simulink model "sequentialProcessorNarenKolli"  (R2018b)
settings: Solver=VariableStepAuto  StartTime=0.0  StopTime=10  RelTol=1e-3
libraries: hdlsllib x172, simulink_extras x9
(part 4 of 4)

== system sequentialProcessorNarenKolli/8-Bit_Processor /8-Bit_Multiplier/First 8-Bit_Adder/Full Adder5/Half Adder ==
  A : Inport
  B : Inport  Port=2
  AND (calculates carry) : Logic  AllPortsSameDT=off  OutDataTypeStr=boolean
  XOR (calculates sum) : Logic  Operator=XOR  AllPortsSameDT=off  OutDataTypeStr=boolean
  Sum : Outport
  Carry : Outport  Port=2
  wires:
  XOR (calculates sum)/1 -> Sum/1
  B/1 -> XOR (calculates sum)/2, AND (calculates carry)/2
  A/1 -> AND (calculates carry)/1, XOR (calculates sum)/1
  AND (calculates carry)/1 -> Carry/1

== system sequentialProcessorNarenKolli/8-Bit_Processor /8-Bit_Multiplier/First 8-Bit_Adder/Full Adder5/Half Adder1 ==
  A : Inport
  B : Inport  Port=2
  AND (calculates carry) : Logic  AllPortsSameDT=off  OutDataTypeStr=boolean
  XOR (calculates sum) : Logic  Operator=XOR  AllPortsSameDT=off  OutDataTypeStr=boolean
  Sum : Outport
  Carry : Outport  Port=2
  wires:
  XOR (calculates sum)/1 -> Sum/1
  B/1 -> XOR (calculates sum)/2, AND (calculates carry)/2
  A/1 -> AND (calculates carry)/1, XOR (calculates sum)/1
  AND (calculates carry)/1 -> Carry/1

== system sequentialProcessorNarenKolli/8-Bit_Processor /8-Bit_Multiplier/First 8-Bit_Adder/Full Adder6/Half Adder ==
  A : Inport
  B : Inport  Port=2
  AND (calculates carry) : Logic  AllPortsSameDT=off  OutDataTypeStr=boolean
  XOR (calculates sum) : Logic  Operator=XOR  AllPortsSameDT=off  OutDataTypeStr=boolean
  Sum : Outport
  Carry : Outport  Port=2
  wires:
  XOR (calculates sum)/1 -> Sum/1
  B/1 -> XOR (calculates sum)/2, AND (calculates carry)/2
  A/1 -> AND (calculates carry)/1, XOR (calculates sum)/1
  AND (calculates carry)/1 -> Carry/1

== system sequentialProcessorNarenKolli/8-Bit_Processor /8-Bit_Multiplier/First 8-Bit_Adder/Full Adder6/Half Adder1 ==
  A : Inport
  B : Inport  Port=2
  AND (calculates carry) : Logic  AllPortsSameDT=off  OutDataTypeStr=boolean
  XOR (calculates sum) : Logic  Operator=XOR  AllPortsSameDT=off  OutDataTypeStr=boolean
  Sum : Outport
  Carry : Outport  Port=2
  wires:
  XOR (calculates sum)/1 -> Sum/1
  B/1 -> XOR (calculates sum)/2, AND (calculates carry)/2
  A/1 -> AND (calculates carry)/1, XOR (calculates sum)/1
  AND (calculates carry)/1 -> Carry/1

== system sequentialProcessorNarenKolli/8-Bit_Processor /8-Bit_Multiplier/First 8-Bit_Adder/Full Adder7/Half Adder ==
  A : Inport
  B : Inport  Port=2
  AND (calculates carry) : Logic  AllPortsSameDT=off  OutDataTypeStr=boolean
  XOR (calculates sum) : Logic  Operator=XOR  AllPortsSameDT=off  OutDataTypeStr=boolean
  Sum : Outport
  Carry : Outport  Port=2
  wires:
  XOR (calculates sum)/1 -> Sum/1
  B/1 -> XOR (calculates sum)/2, AND (calculates carry)/2
  A/1 -> AND (calculates carry)/1, XOR (calculates sum)/1
  AND (calculates carry)/1 -> Carry/1

== system sequentialProcessorNarenKolli/8-Bit_Processor /8-Bit_Multiplier/First 8-Bit_Adder/Full Adder7/Half Adder1 ==
  A : Inport
  B : Inport  Port=2
  AND (calculates carry) : Logic  AllPortsSameDT=off  OutDataTypeStr=boolean
  XOR (calculates sum) : Logic  Operator=XOR  AllPortsSameDT=off  OutDataTypeStr=boolean
  Sum : Outport
  Carry : Outport  Port=2
  wires:
  XOR (calculates sum)/1 -> Sum/1
  B/1 -> XOR (calculates sum)/2, AND (calculates carry)/2
  A/1 -> AND (calculates carry)/1, XOR (calculates sum)/1
  AND (calculates carry)/1 -> Carry/1

== system sequentialProcessorNarenKolli/8-Bit_Processor /8-Bit_Multiplier/Second 4x4 Multiplier/Full Adder/Half Adder ==
  A : Inport
  B : Inport  Port=2
  AND (calculates carry) : Logic  AllPortsSameDT=off  OutDataTypeStr=boolean
  XOR (calculates sum) : Logic  Operator=XOR  AllPortsSameDT=off  OutDataTypeStr=boolean
  Sum : Outport
  Carry : Outport  Port=2
  wires:
  XOR (calculates sum)/1 -> Sum/1
  B/1 -> XOR (calculates sum)/2, AND (calculates carry)/2
  A/1 -> AND (calculates carry)/1, XOR (calculates sum)/1
  AND (calculates carry)/1 -> Carry/1

== system sequentialProcessorNarenKolli/8-Bit_Processor /8-Bit_Multiplier/Second 4x4 Multiplier/Full Adder/Half Adder1 ==
  A : Inport
  B : Inport  Port=2
  AND (calculates carry) : Logic  AllPortsSameDT=off  OutDataTypeStr=boolean
  XOR (calculates sum) : Logic  Operator=XOR  AllPortsSameDT=off  OutDataTypeStr=boolean
  Sum : Outport
  Carry : Outport  Port=2
  wires:
  XOR (calculates sum)/1 -> Sum/1
  B/1 -> XOR (calculates sum)/2, AND (calculates carry)/2
  A/1 -> AND (calculates carry)/1, XOR (calculates sum)/1
  AND (calculates carry)/1 -> Carry/1

== system sequentialProcessorNarenKolli/8-Bit_Processor /8-Bit_Multiplier/Second 4x4 Multiplier/Full Adder1/Half Adder ==
  A : Inport
  B : Inport  Port=2
  AND (calculates carry) : Logic  AllPortsSameDT=off  OutDataTypeStr=boolean
  XOR (calculates sum) : Logic  Operator=XOR  AllPortsSameDT=off  OutDataTypeStr=boolean
  Sum : Outport
  Carry : Outport  Port=2
  wires:
  XOR (calculates sum)/1 -> Sum/1
  B/1 -> XOR (calculates sum)/2, AND (calculates carry)/2
  A/1 -> AND (calculates carry)/1, XOR (calculates sum)/1
  AND (calculates carry)/1 -> Carry/1

== system sequentialProcessorNarenKolli/8-Bit_Processor /8-Bit_Multiplier/Second 4x4 Multiplier/Full Adder1/Half Adder1 ==
  A : Inport
  B : Inport  Port=2
  AND (calculates carry) : Logic  AllPortsSameDT=off  OutDataTypeStr=boolean
  XOR (calculates sum) : Logic  Operator=XOR  AllPortsSameDT=off  OutDataTypeStr=boolean
  Sum : Outport
  Carry : Outport  Port=2
  wires:
  XOR (calculates sum)/1 -> Sum/1
  B/1 -> XOR (calculates sum)/2, AND (calculates carry)/2
  A/1 -> AND (calculates carry)/1, XOR (calculates sum)/1
  AND (calculates carry)/1 -> Carry/1

== system sequentialProcessorNarenKolli/8-Bit_Processor /8-Bit_Multiplier/Second 4x4 Multiplier/Full Adder2/Half Adder ==
  A : Inport
  B : Inport  Port=2
  AND (calculates carry) : Logic  AllPortsSameDT=off  OutDataTypeStr=boolean
  XOR (calculates sum) : Logic  Operator=XOR  AllPortsSameDT=off  OutDataTypeStr=boolean
  Sum : Outport
  Carry : Outport  Port=2
  wires:
  XOR (calculates sum)/1 -> Sum/1
  B/1 -> XOR (calculates sum)/2, AND (calculates carry)/2
  A/1 -> AND (calculates carry)/1, XOR (calculates sum)/1
  AND (calculates carry)/1 -> Carry/1

== system sequentialProcessorNarenKolli/8-Bit_Processor /8-Bit_Multiplier/Second 4x4 Multiplier/Full Adder2/Half Adder1 ==
  A : Inport
  B : Inport  Port=2
  AND (calculates carry) : Logic  AllPortsSameDT=off  OutDataTypeStr=boolean
  XOR (calculates sum) : Logic  Operator=XOR  AllPortsSameDT=off  OutDataTypeStr=boolean
  Sum : Outport
  Carry : Outport  Port=2
  wires:
  XOR (calculates sum)/1 -> Sum/1
  B/1 -> XOR (calculates sum)/2, AND (calculates carry)/2
  A/1 -> AND (calculates carry)/1, XOR (calculates sum)/1
  AND (calculates carry)/1 -> Carry/1

== system sequentialProcessorNarenKolli/8-Bit_Processor /8-Bit_Multiplier/Second 4x4 Multiplier/Full Adder3/Half Adder ==
  A : Inport
  B : Inport  Port=2
  AND (calculates carry) : Logic  AllPortsSameDT=off  OutDataTypeStr=boolean
  XOR (calculates sum) : Logic  Operator=XOR  AllPortsSameDT=off  OutDataTypeStr=boolean
  Sum : Outport
  Carry : Outport  Port=2
  wires:
  XOR (calculates sum)/1 -> Sum/1
  B/1 -> XOR (calculates sum)/2, AND (calculates carry)/2
  A/1 -> AND (calculates carry)/1, XOR (calculates sum)/1
  AND (calculates carry)/1 -> Carry/1

== system sequentialProcessorNarenKolli/8-Bit_Processor /8-Bit_Multiplier/Second 4x4 Multiplier/Full Adder3/Half Adder1 ==
  A : Inport
  B : Inport  Port=2
  AND (calculates carry) : Logic  AllPortsSameDT=off  OutDataTypeStr=boolean
  XOR (calculates sum) : Logic  Operator=XOR  AllPortsSameDT=off  OutDataTypeStr=boolean
  Sum : Outport
  Carry : Outport  Port=2
  wires:
  XOR (calculates sum)/1 -> Sum/1
  B/1 -> XOR (calculates sum)/2, AND (calculates carry)/2
  A/1 -> AND (calculates carry)/1, XOR (calculates sum)/1
  AND (calculates carry)/1 -> Carry/1

== system sequentialProcessorNarenKolli/8-Bit_Processor /8-Bit_Multiplier/Second 4x4 Multiplier/Full Adder4/Half Adder ==
  A : Inport
  B : Inport  Port=2
  AND (calculates carry) : Logic  AllPortsSameDT=off  OutDataTypeStr=boolean
  XOR (calculates sum) : Logic  Operator=XOR  AllPortsSameDT=off  OutDataTypeStr=boolean
  Sum : Outport
  Carry : Outport  Port=2
  wires:
  XOR (calculates sum)/1 -> Sum/1
  B/1 -> XOR (calculates sum)/2, AND (calculates carry)/2
  A/1 -> AND (calculates carry)/1, XOR (calculates sum)/1
  AND (calculates carry)/1 -> Carry/1

== system sequentialProcessorNarenKolli/8-Bit_Processor /8-Bit_Multiplier/Second 4x4 Multiplier/Full Adder4/Half Adder1 ==
  A : Inport
  B : Inport  Port=2
  AND (calculates carry) : Logic  AllPortsSameDT=off  OutDataTypeStr=boolean
  XOR (calculates sum) : Logic  Operator=XOR  AllPortsSameDT=off  OutDataTypeStr=boolean
  Sum : Outport
  Carry : Outport  Port=2
  wires:
  XOR (calculates sum)/1 -> Sum/1
  B/1 -> XOR (calculates sum)/2, AND (calculates carry)/2
  A/1 -> AND (calculates carry)/1, XOR (calculates sum)/1
  AND (calculates carry)/1 -> Carry/1

== system sequentialProcessorNarenKolli/8-Bit_Processor /8-Bit_Multiplier/Second 4x4 Multiplier/Full Adder5/Half Adder ==
  A : Inport
  B : Inport  Port=2
  AND (calculates carry) : Logic  AllPortsSameDT=off  OutDataTypeStr=boolean
  XOR (calculates sum) : Logic  Operator=XOR  AllPortsSameDT=off  OutDataTypeStr=boolean
  Sum : Outport
  Carry : Outport  Port=2
  wires:
  XOR (calculates sum)/1 -> Sum/1
  B/1 -> XOR (calculates sum)/2, AND (calculates carry)/2
  A/1 -> AND (calculates carry)/1, XOR (calculates sum)/1
  AND (calculates carry)/1 -> Carry/1

== system sequentialProcessorNarenKolli/8-Bit_Processor /8-Bit_Multiplier/Second 4x4 Multiplier/Full Adder5/Half Adder1 ==
  A : Inport
  B : Inport  Port=2
  AND (calculates carry) : Logic  AllPortsSameDT=off  OutDataTypeStr=boolean
  XOR (calculates sum) : Logic  Operator=XOR  AllPortsSameDT=off  OutDataTypeStr=boolean
  Sum : Outport
  Carry : Outport  Port=2
  wires:
  XOR (calculates sum)/1 -> Sum/1
  B/1 -> XOR (calculates sum)/2, AND (calculates carry)/2
  A/1 -> AND (calculates carry)/1, XOR (calculates sum)/1
  AND (calculates carry)/1 -> Carry/1

== system sequentialProcessorNarenKolli/8-Bit_Processor /8-Bit_Multiplier/Second 4x4 Multiplier/Full Adder6/Half Adder ==
  A : Inport
  B : Inport  Port=2
  AND (calculates carry) : Logic  AllPortsSameDT=off  OutDataTypeStr=boolean
  XOR (calculates sum) : Logic  Operator=XOR  AllPortsSameDT=off  OutDataTypeStr=boolean
  Sum : Outport
  Carry : Outport  Port=2
  wires:
  XOR (calculates sum)/1 -> Sum/1
  B/1 -> XOR (calculates sum)/2, AND (calculates carry)/2
  A/1 -> AND (calculates carry)/1, XOR (calculates sum)/1
  AND (calculates carry)/1 -> Carry/1

== system sequentialProcessorNarenKolli/8-Bit_Processor /8-Bit_Multiplier/Second 4x4 Multiplier/Full Adder6/Half Adder1 ==
  A : Inport
  B : Inport  Port=2
  AND (calculates carry) : Logic  AllPortsSameDT=off  OutDataTypeStr=boolean
  XOR (calculates sum) : Logic  Operator=XOR  AllPortsSameDT=off  OutDataTypeStr=boolean
  Sum : Outport
  Carry : Outport  Port=2
  wires:
  XOR (calculates sum)/1 -> Sum/1
  B/1 -> XOR (calculates sum)/2, AND (calculates carry)/2
  A/1 -> AND (calculates carry)/1, XOR (calculates sum)/1
  AND (calculates carry)/1 -> Carry/1

== system sequentialProcessorNarenKolli/8-Bit_Processor /8-Bit_Multiplier/Second 4x4 Multiplier/Full Adder7/Half Adder ==
  A : Inport
  B : Inport  Port=2
  AND (calculates carry) : Logic  AllPortsSameDT=off  OutDataTypeStr=boolean
  XOR (calculates sum) : Logic  Operator=XOR  AllPortsSameDT=off  OutDataTypeStr=boolean
  Sum : Outport
  Carry : Outport  Port=2
  wires:
  XOR (calculates sum)/1 -> Sum/1
  B/1 -> XOR (calculates sum)/2, AND (calculates carry)/2
  A/1 -> AND (calculates carry)/1, XOR (calculates sum)/1
  AND (calculates carry)/1 -> Carry/1

== system sequentialProcessorNarenKolli/8-Bit_Processor /8-Bit_Multiplier/Second 4x4 Multiplier/Full Adder7/Half Adder1 ==
  A : Inport
  B : Inport  Port=2
  AND (calculates carry) : Logic  AllPortsSameDT=off  OutDataTypeStr=boolean
  XOR (calculates sum) : Logic  Operator=XOR  AllPortsSameDT=off  OutDataTypeStr=boolean
  Sum : Outport
  Carry : Outport  Port=2
  wires:
  XOR (calculates sum)/1 -> Sum/1
  B/1 -> XOR (calculates sum)/2, AND (calculates carry)/2
  A/1 -> AND (calculates carry)/1, XOR (calculates sum)/1
  AND (calculates carry)/1 -> Carry/1

== system sequentialProcessorNarenKolli/8-Bit_Processor /8-Bit_Multiplier/Second 8-Bit_Adder1/Full Adder/Half Adder ==
  A : Inport
  B : Inport  Port=2
  AND (calculates carry) : Logic  AllPortsSameDT=off  OutDataTypeStr=boolean
  XOR (calculates sum) : Logic  Operator=XOR  AllPortsSameDT=off  OutDataTypeStr=boolean
  Sum : Outport
  Carry : Outport  Port=2
  wires:
  XOR (calculates sum)/1 -> Sum/1
  B/1 -> XOR (calculates sum)/2, AND (calculates carry)/2
  A/1 -> AND (calculates carry)/1, XOR (calculates sum)/1
  AND (calculates carry)/1 -> Carry/1

== system sequentialProcessorNarenKolli/8-Bit_Processor /8-Bit_Multiplier/Second 8-Bit_Adder1/Full Adder/Half Adder1 ==
  A : Inport
  B : Inport  Port=2
  AND (calculates carry) : Logic  AllPortsSameDT=off  OutDataTypeStr=boolean
  XOR (calculates sum) : Logic  Operator=XOR  AllPortsSameDT=off  OutDataTypeStr=boolean
  Sum : Outport
  Carry : Outport  Port=2
  wires:
  XOR (calculates sum)/1 -> Sum/1
  B/1 -> XOR (calculates sum)/2, AND (calculates carry)/2
  A/1 -> AND (calculates carry)/1, XOR (calculates sum)/1
  AND (calculates carry)/1 -> Carry/1

== system sequentialProcessorNarenKolli/8-Bit_Processor /8-Bit_Multiplier/Second 8-Bit_Adder1/Full Adder1/Half Adder ==
  A : Inport
  B : Inport  Port=2
  AND (calculates carry) : Logic  AllPortsSameDT=off  OutDataTypeStr=boolean
  XOR (calculates sum) : Logic  Operator=XOR  AllPortsSameDT=off  OutDataTypeStr=boolean
  Sum : Outport
  Carry : Outport  Port=2
  wires:
  XOR (calculates sum)/1 -> Sum/1
  B/1 -> XOR (calculates sum)/2, AND (calculates carry)/2
  A/1 -> AND (calculates carry)/1, XOR (calculates sum)/1
  AND (calculates carry)/1 -> Carry/1

== system sequentialProcessorNarenKolli/8-Bit_Processor /8-Bit_Multiplier/Second 8-Bit_Adder1/Full Adder1/Half Adder1 ==
  A : Inport
  B : Inport  Port=2
  AND (calculates carry) : Logic  AllPortsSameDT=off  OutDataTypeStr=boolean
  XOR (calculates sum) : Logic  Operator=XOR  AllPortsSameDT=off  OutDataTypeStr=boolean
  Sum : Outport
  Carry : Outport  Port=2
  wires:
  XOR (calculates sum)/1 -> Sum/1
  B/1 -> XOR (calculates sum)/2, AND (calculates carry)/2
  A/1 -> AND (calculates carry)/1, XOR (calculates sum)/1
  AND (calculates carry)/1 -> Carry/1

== system sequentialProcessorNarenKolli/8-Bit_Processor /8-Bit_Multiplier/Second 8-Bit_Adder1/Full Adder2/Half Adder ==
  A : Inport
  B : Inport  Port=2
  AND (calculates carry) : Logic  AllPortsSameDT=off  OutDataTypeStr=boolean
  XOR (calculates sum) : Logic  Operator=XOR  AllPortsSameDT=off  OutDataTypeStr=boolean
  Sum : Outport
  Carry : Outport  Port=2
  wires:
  XOR (calculates sum)/1 -> Sum/1
  B/1 -> XOR (calculates sum)/2, AND (calculates carry)/2
  A/1 -> AND (calculates carry)/1, XOR (calculates sum)/1
  AND (calculates carry)/1 -> Carry/1

== system sequentialProcessorNarenKolli/8-Bit_Processor /8-Bit_Multiplier/Second 8-Bit_Adder1/Full Adder2/Half Adder1 ==
  A : Inport
  B : Inport  Port=2
  AND (calculates carry) : Logic  AllPortsSameDT=off  OutDataTypeStr=boolean
  XOR (calculates sum) : Logic  Operator=XOR  AllPortsSameDT=off  OutDataTypeStr=boolean
  Sum : Outport
  Carry : Outport  Port=2
  wires:
  XOR (calculates sum)/1 -> Sum/1
  B/1 -> XOR (calculates sum)/2, AND (calculates carry)/2
  A/1 -> AND (calculates carry)/1, XOR (calculates sum)/1
  AND (calculates carry)/1 -> Carry/1

== system sequentialProcessorNarenKolli/8-Bit_Processor /8-Bit_Multiplier/Second 8-Bit_Adder1/Full Adder3/Half Adder ==
  A : Inport
  B : Inport  Port=2
  AND (calculates carry) : Logic  AllPortsSameDT=off  OutDataTypeStr=boolean
  XOR (calculates sum) : Logic  Operator=XOR  AllPortsSameDT=off  OutDataTypeStr=boolean
  Sum : Outport
  Carry : Outport  Port=2
  wires:
  XOR (calculates sum)/1 -> Sum/1
  B/1 -> XOR (calculates sum)/2, AND (calculates carry)/2
  A/1 -> AND (calculates carry)/1, XOR (calculates sum)/1
  AND (calculates carry)/1 -> Carry/1

== system sequentialProcessorNarenKolli/8-Bit_Processor /8-Bit_Multiplier/Second 8-Bit_Adder1/Full Adder3/Half Adder1 ==
  A : Inport
  B : Inport  Port=2
  AND (calculates carry) : Logic  AllPortsSameDT=off  OutDataTypeStr=boolean
  XOR (calculates sum) : Logic  Operator=XOR  AllPortsSameDT=off  OutDataTypeStr=boolean
  Sum : Outport
  Carry : Outport  Port=2
  wires:
  XOR (calculates sum)/1 -> Sum/1
  B/1 -> XOR (calculates sum)/2, AND (calculates carry)/2
  A/1 -> AND (calculates carry)/1, XOR (calculates sum)/1
  AND (calculates carry)/1 -> Carry/1

== system sequentialProcessorNarenKolli/8-Bit_Processor /8-Bit_Multiplier/Second 8-Bit_Adder1/Full Adder4/Half Adder ==
  A : Inport
  B : Inport  Port=2
  AND (calculates carry) : Logic  AllPortsSameDT=off  OutDataTypeStr=boolean
  XOR (calculates sum) : Logic  Operator=XOR  AllPortsSameDT=off  OutDataTypeStr=boolean
  Sum : Outport
  Carry : Outport  Port=2
  wires:
  XOR (calculates sum)/1 -> Sum/1
  B/1 -> XOR (calculates sum)/2, AND (calculates carry)/2
  A/1 -> AND (calculates carry)/1, XOR (calculates sum)/1
  AND (calculates carry)/1 -> Carry/1

== system sequentialProcessorNarenKolli/8-Bit_Processor /8-Bit_Multiplier/Second 8-Bit_Adder1/Full Adder4/Half Adder1 ==
  A : Inport
  B : Inport  Port=2
  AND (calculates carry) : Logic  AllPortsSameDT=off  OutDataTypeStr=boolean
  XOR (calculates sum) : Logic  Operator=XOR  AllPortsSameDT=off  OutDataTypeStr=boolean
  Sum : Outport
  Carry : Outport  Port=2
  wires:
  XOR (calculates sum)/1 -> Sum/1
  B/1 -> XOR (calculates sum)/2, AND (calculates carry)/2
  A/1 -> AND (calculates carry)/1, XOR (calculates sum)/1
  AND (calculates carry)/1 -> Carry/1

== system sequentialProcessorNarenKolli/8-Bit_Processor /8-Bit_Multiplier/Second 8-Bit_Adder1/Full Adder5/Half Adder ==
  A : Inport
  B : Inport  Port=2
  AND (calculates carry) : Logic  AllPortsSameDT=off  OutDataTypeStr=boolean
  XOR (calculates sum) : Logic  Operator=XOR  AllPortsSameDT=off  OutDataTypeStr=boolean
  Sum : Outport
  Carry : Outport  Port=2
  wires:
  XOR (calculates sum)/1 -> Sum/1
  B/1 -> XOR (calculates sum)/2, AND (calculates carry)/2
  A/1 -> AND (calculates carry)/1, XOR (calculates sum)/1
  AND (calculates carry)/1 -> Carry/1

== system sequentialProcessorNarenKolli/8-Bit_Processor /8-Bit_Multiplier/Second 8-Bit_Adder1/Full Adder5/Half Adder1 ==
  A : Inport
  B : Inport  Port=2
  AND (calculates carry) : Logic  AllPortsSameDT=off  OutDataTypeStr=boolean
  XOR (calculates sum) : Logic  Operator=XOR  AllPortsSameDT=off  OutDataTypeStr=boolean
  Sum : Outport
  Carry : Outport  Port=2
  wires:
  XOR (calculates sum)/1 -> Sum/1
  B/1 -> XOR (calculates sum)/2, AND (calculates carry)/2
  A/1 -> AND (calculates carry)/1, XOR (calculates sum)/1
  AND (calculates carry)/1 -> Carry/1

== system sequentialProcessorNarenKolli/8-Bit_Processor /8-Bit_Multiplier/Second 8-Bit_Adder1/Full Adder6/Half Adder ==
  A : Inport
  B : Inport  Port=2
  AND (calculates carry) : Logic  AllPortsSameDT=off  OutDataTypeStr=boolean
  XOR (calculates sum) : Logic  Operator=XOR  AllPortsSameDT=off  OutDataTypeStr=boolean
  Sum : Outport
  Carry : Outport  Port=2
  wires:
  XOR (calculates sum)/1 -> Sum/1
  B/1 -> XOR (calculates sum)/2, AND (calculates carry)/2
  A/1 -> AND (calculates carry)/1, XOR (calculates sum)/1
  AND (calculates carry)/1 -> Carry/1

== system sequentialProcessorNarenKolli/8-Bit_Processor /8-Bit_Multiplier/Second 8-Bit_Adder1/Full Adder6/Half Adder1 ==
  A : Inport
  B : Inport  Port=2
  AND (calculates carry) : Logic  AllPortsSameDT=off  OutDataTypeStr=boolean
  XOR (calculates sum) : Logic  Operator=XOR  AllPortsSameDT=off  OutDataTypeStr=boolean
  Sum : Outport
  Carry : Outport  Port=2
  wires:
  XOR (calculates sum)/1 -> Sum/1
  B/1 -> XOR (calculates sum)/2, AND (calculates carry)/2
  A/1 -> AND (calculates carry)/1, XOR (calculates sum)/1
  AND (calculates carry)/1 -> Carry/1

== system sequentialProcessorNarenKolli/8-Bit_Processor /8-Bit_Multiplier/Second 8-Bit_Adder1/Full Adder7/Half Adder ==
  A : Inport
  B : Inport  Port=2
  AND (calculates carry) : Logic  AllPortsSameDT=off  OutDataTypeStr=boolean
  XOR (calculates sum) : Logic  Operator=XOR  AllPortsSameDT=off  OutDataTypeStr=boolean
  Sum : Outport
  Carry : Outport  Port=2
  wires:
  XOR (calculates sum)/1 -> Sum/1
  B/1 -> XOR (calculates sum)/2, AND (calculates carry)/2
  A/1 -> AND (calculates carry)/1, XOR (calculates sum)/1
  AND (calculates carry)/1 -> Carry/1

== system sequentialProcessorNarenKolli/8-Bit_Processor /8-Bit_Multiplier/Second 8-Bit_Adder1/Full Adder7/Half Adder1 ==
  A : Inport
  B : Inport  Port=2
  AND (calculates carry) : Logic  AllPortsSameDT=off  OutDataTypeStr=boolean
  XOR (calculates sum) : Logic  Operator=XOR  AllPortsSameDT=off  OutDataTypeStr=boolean
  Sum : Outport
  Carry : Outport  Port=2
  wires:
  XOR (calculates sum)/1 -> Sum/1
  B/1 -> XOR (calculates sum)/2, AND (calculates carry)/2
  A/1 -> AND (calculates carry)/1, XOR (calculates sum)/1
  AND (calculates carry)/1 -> Carry/1

== system sequentialProcessorNarenKolli/8-Bit_Processor /8-Bit_Multiplier/Third 4x4 Multiplier/Full Adder/Half Adder ==
  A : Inport
  B : Inport  Port=2
  AND (calculates carry) : Logic  AllPortsSameDT=off  OutDataTypeStr=boolean
  XOR (calculates sum) : Logic  Operator=XOR  AllPortsSameDT=off  OutDataTypeStr=boolean
  Sum : Outport
  Carry : Outport  Port=2
  wires:
  XOR (calculates sum)/1 -> Sum/1
  B/1 -> XOR (calculates sum)/2, AND (calculates carry)/2
  A/1 -> AND (calculates carry)/1, XOR (calculates sum)/1
  AND (calculates carry)/1 -> Carry/1

== system sequentialProcessorNarenKolli/8-Bit_Processor /8-Bit_Multiplier/Third 4x4 Multiplier/Full Adder/Half Adder1 ==
  A : Inport
  B : Inport  Port=2
  AND (calculates carry) : Logic  AllPortsSameDT=off  OutDataTypeStr=boolean
  XOR (calculates sum) : Logic  Operator=XOR  AllPortsSameDT=off  OutDataTypeStr=boolean
  Sum : Outport
  Carry : Outport  Port=2
  wires:
  XOR (calculates sum)/1 -> Sum/1
  B/1 -> XOR (calculates sum)/2, AND (calculates carry)/2
  A/1 -> AND (calculates carry)/1, XOR (calculates sum)/1
  AND (calculates carry)/1 -> Carry/1

== system sequentialProcessorNarenKolli/8-Bit_Processor /8-Bit_Multiplier/Third 4x4 Multiplier/Full Adder1/Half Adder ==
  A : Inport
  B : Inport  Port=2
  AND (calculates carry) : Logic  AllPortsSameDT=off  OutDataTypeStr=boolean
  XOR (calculates sum) : Logic  Operator=XOR  AllPortsSameDT=off  OutDataTypeStr=boolean
  Sum : Outport
  Carry : Outport  Port=2
  wires:
  XOR (calculates sum)/1 -> Sum/1
  B/1 -> XOR (calculates sum)/2, AND (calculates carry)/2
  A/1 -> AND (calculates carry)/1, XOR (calculates sum)/1
  AND (calculates carry)/1 -> Carry/1

== system sequentialProcessorNarenKolli/8-Bit_Processor /8-Bit_Multiplier/Third 4x4 Multiplier/Full Adder1/Half Adder1 ==
  A : Inport
  B : Inport  Port=2
  AND (calculates carry) : Logic  AllPortsSameDT=off  OutDataTypeStr=boolean
  XOR (calculates sum) : Logic  Operator=XOR  AllPortsSameDT=off  OutDataTypeStr=boolean
  Sum : Outport
  Carry : Outport  Port=2
  wires:
  XOR (calculates sum)/1 -> Sum/1
  B/1 -> XOR (calculates sum)/2, AND (calculates carry)/2
  A/1 -> AND (calculates carry)/1, XOR (calculates sum)/1
  AND (calculates carry)/1 -> Carry/1

== system sequentialProcessorNarenKolli/8-Bit_Processor /8-Bit_Multiplier/Third 4x4 Multiplier/Full Adder2/Half Adder ==
  A : Inport
  B : Inport  Port=2
  AND (calculates carry) : Logic  AllPortsSameDT=off  OutDataTypeStr=boolean
  XOR (calculates sum) : Logic  Operator=XOR  AllPortsSameDT=off  OutDataTypeStr=boolean
  Sum : Outport
  Carry : Outport  Port=2
  wires:
  XOR (calculates sum)/1 -> Sum/1
  B/1 -> XOR (calculates sum)/2, AND (calculates carry)/2
  A/1 -> AND (calculates carry)/1, XOR (calculates sum)/1
  AND (calculates carry)/1 -> Carry/1

== system sequentialProcessorNarenKolli/8-Bit_Processor /8-Bit_Multiplier/Third 4x4 Multiplier/Full Adder2/Half Adder1 ==
  A : Inport
  B : Inport  Port=2
  AND (calculates carry) : Logic  AllPortsSameDT=off  OutDataTypeStr=boolean
  XOR (calculates sum) : Logic  Operator=XOR  AllPortsSameDT=off  OutDataTypeStr=boolean
  Sum : Outport
  Carry : Outport  Port=2
  wires:
  XOR (calculates sum)/1 -> Sum/1
  B/1 -> XOR (calculates sum)/2, AND (calculates carry)/2
  A/1 -> AND (calculates carry)/1, XOR (calculates sum)/1
  AND (calculates carry)/1 -> Carry/1

== system sequentialProcessorNarenKolli/8-Bit_Processor /8-Bit_Multiplier/Third 4x4 Multiplier/Full Adder3/Half Adder ==
  A : Inport
  B : Inport  Port=2
  AND (calculates carry) : Logic  AllPortsSameDT=off  OutDataTypeStr=boolean
  XOR (calculates sum) : Logic  Operator=XOR  AllPortsSameDT=off  OutDataTypeStr=boolean
  Sum : Outport
  Carry : Outport  Port=2
  wires:
  XOR (calculates sum)/1 -> Sum/1
  B/1 -> XOR (calculates sum)/2, AND (calculates carry)/2
  A/1 -> AND (calculates carry)/1, XOR (calculates sum)/1
  AND (calculates carry)/1 -> Carry/1

== system sequentialProcessorNarenKolli/8-Bit_Processor /8-Bit_Multiplier/Third 4x4 Multiplier/Full Adder3/Half Adder1 ==
  A : Inport
  B : Inport  Port=2
  AND (calculates carry) : Logic  AllPortsSameDT=off  OutDataTypeStr=boolean
  XOR (calculates sum) : Logic  Operator=XOR  AllPortsSameDT=off  OutDataTypeStr=boolean
  Sum : Outport
  Carry : Outport  Port=2
  wires:
  XOR (calculates sum)/1 -> Sum/1
  B/1 -> XOR (calculates sum)/2, AND (calculates carry)/2
  A/1 -> AND (calculates carry)/1, XOR (calculates sum)/1
  AND (calculates carry)/1 -> Carry/1

== system sequentialProcessorNarenKolli/8-Bit_Processor /8-Bit_Multiplier/Third 4x4 Multiplier/Full Adder4/Half Adder ==
  A : Inport
  B : Inport  Port=2
  AND (calculates carry) : Logic  AllPortsSameDT=off  OutDataTypeStr=boolean
  XOR (calculates sum) : Logic  Operator=XOR  AllPortsSameDT=off  OutDataTypeStr=boolean
  Sum : Outport
  Carry : Outport  Port=2
  wires:
  XOR (calculates sum)/1 -> Sum/1
  B/1 -> XOR (calculates sum)/2, AND (calculates carry)/2
  A/1 -> AND (calculates carry)/1, XOR (calculates sum)/1
  AND (calculates carry)/1 -> Carry/1

== system sequentialProcessorNarenKolli/8-Bit_Processor /8-Bit_Multiplier/Third 4x4 Multiplier/Full Adder4/Half Adder1 ==
  A : Inport
  B : Inport  Port=2
  AND (calculates carry) : Logic  AllPortsSameDT=off  OutDataTypeStr=boolean
  XOR (calculates sum) : Logic  Operator=XOR  AllPortsSameDT=off  OutDataTypeStr=boolean
  Sum : Outport
  Carry : Outport  Port=2
  wires:
  XOR (calculates sum)/1 -> Sum/1
  B/1 -> XOR (calculates sum)/2, AND (calculates carry)/2
  A/1 -> AND (calculates carry)/1, XOR (calculates sum)/1
  AND (calculates carry)/1 -> Carry/1

== system sequentialProcessorNarenKolli/8-Bit_Processor /8-Bit_Multiplier/Third 4x4 Multiplier/Full Adder5/Half Adder ==
  A : Inport
  B : Inport  Port=2
  AND (calculates carry) : Logic  AllPortsSameDT=off  OutDataTypeStr=boolean
  XOR (calculates sum) : Logic  Operator=XOR  AllPortsSameDT=off  OutDataTypeStr=boolean
  Sum : Outport
  Carry : Outport  Port=2
  wires:
  XOR (calculates sum)/1 -> Sum/1
  B/1 -> XOR (calculates sum)/2, AND (calculates carry)/2
  A/1 -> AND (calculates carry)/1, XOR (calculates sum)/1
  AND (calculates carry)/1 -> Carry/1

== system sequentialProcessorNarenKolli/8-Bit_Processor /8-Bit_Multiplier/Third 4x4 Multiplier/Full Adder5/Half Adder1 ==
  A : Inport
  B : Inport  Port=2
  AND (calculates carry) : Logic  AllPortsSameDT=off  OutDataTypeStr=boolean
  XOR (calculates sum) : Logic  Operator=XOR  AllPortsSameDT=off  OutDataTypeStr=boolean
  Sum : Outport
  Carry : Outport  Port=2
  wires:
  XOR (calculates sum)/1 -> Sum/1
  B/1 -> XOR (calculates sum)/2, AND (calculates carry)/2
  A/1 -> AND (calculates carry)/1, XOR (calculates sum)/1
  AND (calculates carry)/1 -> Carry/1

== system sequentialProcessorNarenKolli/8-Bit_Processor /8-Bit_Multiplier/Third 4x4 Multiplier/Full Adder6/Half Adder ==
  A : Inport
  B : Inport  Port=2
  AND (calculates carry) : Logic  AllPortsSameDT=off  OutDataTypeStr=boolean
  XOR (calculates sum) : Logic  Operator=XOR  AllPortsSameDT=off  OutDataTypeStr=boolean
  Sum : Outport
  Carry : Outport  Port=2
  wires:
  XOR (calculates sum)/1 -> Sum/1
  B/1 -> XOR (calculates sum)/2, AND (calculates carry)/2
  A/1 -> AND (calculates carry)/1, XOR (calculates sum)/1
  AND (calculates carry)/1 -> Carry/1

== system sequentialProcessorNarenKolli/8-Bit_Processor /8-Bit_Multiplier/Third 4x4 Multiplier/Full Adder6/Half Adder1 ==
  A : Inport
  B : Inport  Port=2
  AND (calculates carry) : Logic  AllPortsSameDT=off  OutDataTypeStr=boolean
  XOR (calculates sum) : Logic  Operator=XOR  AllPortsSameDT=off  OutDataTypeStr=boolean
  Sum : Outport
  Carry : Outport  Port=2
  wires:
  XOR (calculates sum)/1 -> Sum/1
  B/1 -> XOR (calculates sum)/2, AND (calculates carry)/2
  A/1 -> AND (calculates carry)/1, XOR (calculates sum)/1
  AND (calculates carry)/1 -> Carry/1

== system sequentialProcessorNarenKolli/8-Bit_Processor /8-Bit_Multiplier/Third 4x4 Multiplier/Full Adder7/Half Adder ==
  A : Inport
  B : Inport  Port=2
  AND (calculates carry) : Logic  AllPortsSameDT=off  OutDataTypeStr=boolean
  XOR (calculates sum) : Logic  Operator=XOR  AllPortsSameDT=off  OutDataTypeStr=boolean
  Sum : Outport
  Carry : Outport  Port=2
  wires:
  XOR (calculates sum)/1 -> Sum/1
  B/1 -> XOR (calculates sum)/2, AND (calculates carry)/2
  A/1 -> AND (calculates carry)/1, XOR (calculates sum)/1
  AND (calculates carry)/1 -> Carry/1

== system sequentialProcessorNarenKolli/8-Bit_Processor /8-Bit_Multiplier/Third 4x4 Multiplier/Full Adder7/Half Adder1 ==
  A : Inport
  B : Inport  Port=2
  AND (calculates carry) : Logic  AllPortsSameDT=off  OutDataTypeStr=boolean
  XOR (calculates sum) : Logic  Operator=XOR  AllPortsSameDT=off  OutDataTypeStr=boolean
  Sum : Outport
  Carry : Outport  Port=2
  wires:
  XOR (calculates sum)/1 -> Sum/1
  B/1 -> XOR (calculates sum)/2, AND (calculates carry)/2
  A/1 -> AND (calculates carry)/1, XOR (calculates sum)/1
  AND (calculates carry)/1 -> Carry/1
